simulink model "Car_Dynamics"  (R2019b)
settings: Solver=VariableStepAuto  StartTime=0.0  StopTime=10.0  RelTol=1e-3
settings Model: Creator=michael  LastModifiedBy=michael

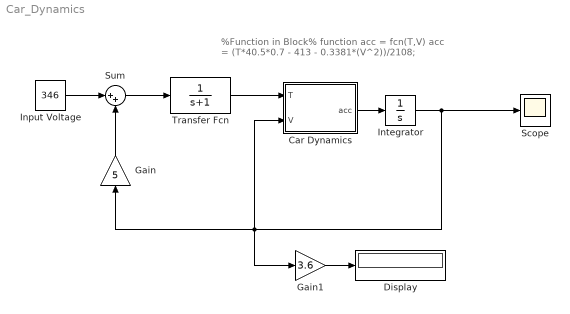
== system Car_Dynamics ==
  note: %Function in Block%
      | function acc = fcn(T,V)
      | acc = (T*40.5*0.7 - 413 - 0.3381*(V^2))/2108;
  Car Dynamics : MATLAB Function  TreatAsAtomicUnit=on
  Display : Display
  Gain : Gain  Gain=5
  Gain1 : Gain  Gain=3.6
  Input Voltage : Constant  Value=346
  Integrator : Integrator
  Scope : Scope
  Sum : Sum  Inputs=|++
  Transfer Fcn : TransferFcn  Denominator=[1 1]
  wires:
  Input Voltage/1 -> Sum/1
  Sum/1 -> Transfer Fcn/1
  Gain/1 -> Sum/2
  Transfer Fcn/1 -> Car Dynamics/1(T)
  Car Dynamics/1(acc) -> Integrator/1
  Integrator/1 -> Scope/1, Gain/1, Gain1/1, Car Dynamics/2(V)
  Gain1/1 -> Display/1

== matlab function Car_Dynamics/Car Dynamics ==
  data: T input; acc output; V input
function acc = fcn(T,V)
acc = (T*40.5*0.7 - 413 - 0.3381*(V^2))/2108;
